simulink model "fir_core_model"  (R2021a)
settings: Solver=FixedStepDiscrete  StartTime=0.0  StopTime=100  FixedStep=1  RelTol=1e-3
settings Model: Creator=user  LastModifiedBy=user

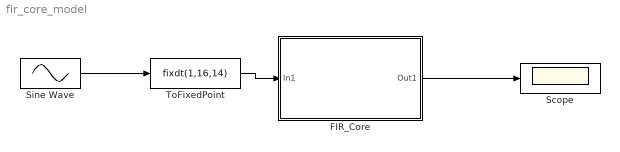
== system fir_core_model ==
  FIR_Core : Subsystem
  Scope : Scope
  Sine Wave : Sin  Frequency=0.05  SampleTime=1
  ToFixedPoint : DataTypeConversion  OutDataTypeStr=fixdt(1,16,14)
  wires:
  Sine Wave/1 -> ToFixedPoint/1
  ToFixedPoint/1 -> FIR_Core/1(In1)
  FIR_Core/1(Out1) -> Scope/1

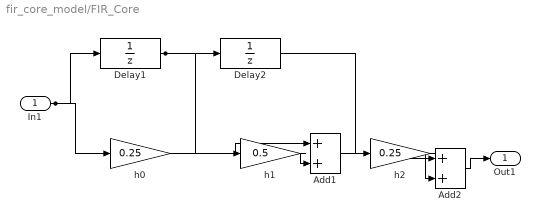
== system fir_core_model/FIR_Core ==
  In1 : Inport
  Add1 : Sum
  Add2 : Sum
  Delay1 : UnitDelay  HasFrameUpgradeWarning=on
  Delay2 : UnitDelay  HasFrameUpgradeWarning=on
  h0 : Gain  Gain=0.25  OutDataTypeStr=fixdt(1,18,14)
  h1 : Gain  Gain=0.5  OutDataTypeStr=fixdt(1,18,14)
  h2 : Gain  Gain=0.25  OutDataTypeStr=fixdt(1,18,14)
  Out1 : Outport
  wires:
  In1/1 -> Delay1/1, h0/1
  Delay1/1 -> Delay2/1, h1/1
  Delay2/1 -> h2/1
  h0/1 -> Add1/1
  h1/1 -> Add1/2
  Add1/1 -> Add2/1
  h2/1 -> Add2/2
  Add2/1 -> Out1/1
